simulink subsystem "BMS_slave"  (R2021a)
settings: Solver=VariableStepAuto  StartTime=0.0  StopTime=10.0  RelTol=1e-3
undefined symbols (not defined in the file): Discharge_Res
libraries: fl_lib x30, nesl_utility x20, ee_lib x10
settings Model: Creator=Carlo Edoardo  LastModifiedBy=Carlo Edoardo

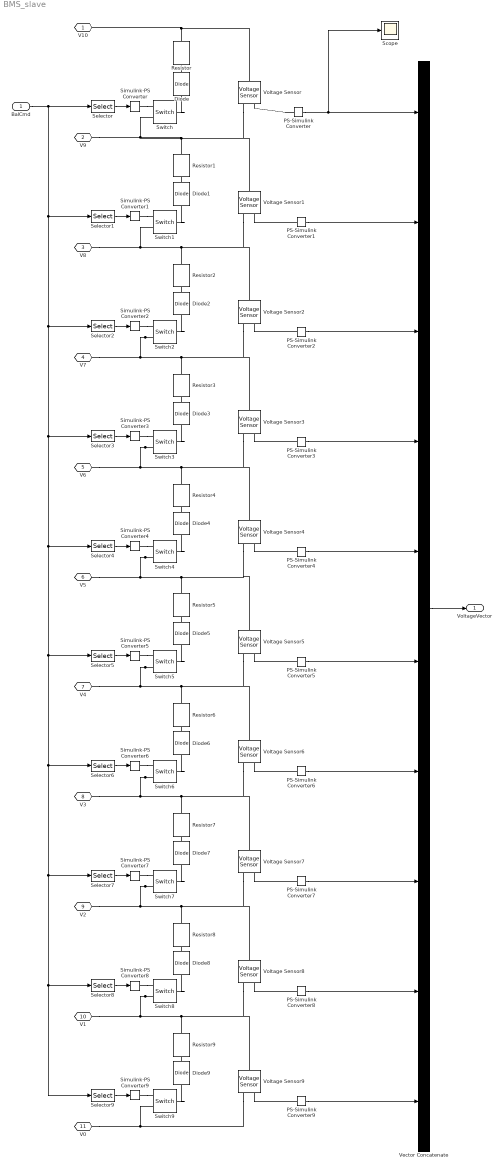
== system BMS_slave ==
  BalCmd : Inport
  Diode{,1..9} (10 alike) : ee_lib/Semiconductors & Converters/Diode  ModelType=ee.enum.diode.modelType.pwl  IfMat=[.07, .12, .19, 1.75, 4.24, 7.32, 11.2; .16, .3, .72, 2.14, 4.02, 6.35, 9.12] A  TjVec=[25, 125] degC  VfVec=[.5, .7, .9, 1.3, 1.7, 2.1, 2.5] V  Vf=0.6 V  Ron=0.3 Ohm  Goff=1e-8 S  prmExp=ee.enum.diode.expParam.useTwo  I12=[.0137, .545] A  V12=[.6, .7] V  IS=1e-12 A  ec=1  I1=0.0137 A  V1=0.6 V  RS=0 Ohm  Tmeas=25 degC  N_series=1  N_parallel=1  Rz=0.3 Ohm  BV=inf V  C_param=ee.enum.diode.capParam.fixed  CJ=5 pF  CJ0=5 pF  VJ=1 V  Mgrad=0.5  Vvec=[.1, 10, 100] V  Cvec=[3.5, 1, .4] pF  FC=0.5  Q_param=ee.enum.diode.recoveryParam.off  iRM=-7.15 A  iF=4 A  didt=-750 A/us  trr_factor=3  trr=115 ns  Qrr=150 s*nA  TT=50 ns  tau=100 ns  T_param=ee.enum.diode.temperatureParam.off  IS_T2=1.25e-7 A  I1_T2=0.245 A  V1_T2=0.5 V  Tmeas2=125 degC  EG_param=ee.enum.diode.egapParam.material_si  EG=1.11 eV  XTI_param=ee.enum.diode.xtiParam.pn  XTI=3  dBVdT=0 V/K  enable_faults=ee.enum.faults.faultEnable.no  fault_action=ee.enum.faults.faultAction.none  fault_types=ee.enum.diode.faults.open  tau_fault=1e-3 s  IfMat_faulted=[.07, .12, .19, 1.75, 4.24, 7.32, 11.2; .16, .3, .72, 2.14, 4.02, 6.35, 9.12] A  VfVec_faulted=[.5, .7, .9, 1.3, 1.7, 2.1, 2.5] V  Ropen_faulted=1000 Ohm  Gshort_faulted=1000 1/Ohm  Vf_faulted=0.6 V  Ron_faulted=0.3 Ohm  Goff_faulted=1e-8 S  I12_faulted=[.0137, .545] A  V12_faulted=[.6, .7] V  IS_faulted=1e-12 A  ec_faulted=1  I1_faulted=0.0137 A  V1_faulted=0.6 V  RS_faulted=0 Ohm  Rz_faulted=0.3 Ohm  BV_faulted=inf V  Cscale_faulted=100  enable_temporal_fault=ee.enum.faults.faultEnable.no  t_fault=inf s  enable_behavioral_fault=ee.enum.faults.faultEnable.no  max_permissible_voltage=inf V  n_fail_on_voltage=1  max_permissible_current=inf A  t_fail_on_current=1 s  max_permissible_dVdt=inf V/s  Tdevice=25 degC  i_specify=off  i_priority=None  i=0 A  i_nominal_specify=off  i_nominal_unit=A  i_nominal_value=1  v_specify=off  v_priority=None  v=0 V  v_nominal_specify=off  v_nominal_unit=V  v_nominal_value=1  i_diode_specify=off  i_diode_priority=None  i_diode=0 A  i_diode_nominal_specify=off  i_diode_nominal_unit=A  i_diode_nominal_value=1  v_diode_specify=off  v_diode_priority=None  v_diode=0 V  v_diode_nominal_specify=off  v_diode_nominal_unit=V  v_diode_nominal_value=1  i_capacitor_specify=off  i_capacitor_priority=None  i_capacitor=0 A  i_capacitor_nominal_specify=off  i_capacitor_nominal_unit=A  i_capacitor_nominal_value=1  v_capacitor_specify=off  v_capacitor_priority=None  v_capacitor=0 V  v_capacitor_nominal_specify=off  v_capacitor_nominal_unit=V  v_capacitor_nominal_value=1  power_dissipated_specify=off  power_dissipated_priority=None  power_dissipated=0 W  power_dissipated_nominal_specify=off  power_dissipated_nominal_unit=W  power_dissipated_nominal_value=1  max_permissible_temperature=inf K  t_fail_on_temperature=1 s  thermal_network_parameterization=ee.enum.thermalNetworkTopology.cauer  Rth=[0, 10] K/W  Rth_Foster=[4, 6] K/W  thermal_mass_parameterization=ee.enum.thermalNetwork.timeconstant  thermal_mass=[0, 1] J/K  thermal_mass_Foster=[1.5, 3] J/K  thermal_time_constant=[0, 10] s  thermal_time_constant_Foster=[6, 18] s  thermal_mass_initial_temperatures=[25, 25] degC
  PS-Simulink Converter{,1..9} (10 alike) : nesl_utility/PS-Simulink Converter  PhysicalDomain=network_engine_domain  SubClassName=ps_output  LeftPortType=input  RightPortType=output  PseudoPeriodic=off  Frequencies=[]  Unit=inherit  AffineConversion=off
      settings: SourceProductBaseCode=PW,SS
  Resistor{,1..9} (10 alike) : fl_lib/Electrical/Electrical Elements/Resistor  R=Discharge_Res Ohm  i_specify=off  i_priority=None  i=0 A  i_nominal_specify=off  i_nominal_unit=A  i_nominal_value=1  v_specify=off  v_priority=None  v=0 V  v_nominal_specify=off  v_nominal_unit=V  v_nominal_value=1
  Scope : Scope
  Selector : Selector  InputPortWidth=10  IndexOptions=Index vector (dialog)  Indices=1  OutputSizes=1
  Selector1 : Selector  InputPortWidth=10  IndexOptions=Index vector (dialog)  Indices=2  OutputSizes=1
  Selector2 : Selector  InputPortWidth=10  IndexOptions=Index vector (dialog)  Indices=3  OutputSizes=1
  Selector3 : Selector  InputPortWidth=10  IndexOptions=Index vector (dialog)  Indices=4  OutputSizes=1
  Selector4 : Selector  InputPortWidth=10  IndexOptions=Index vector (dialog)  Indices=5  OutputSizes=1
  Selector5 : Selector  InputPortWidth=10  IndexOptions=Index vector (dialog)  Indices=6  OutputSizes=1
  Selector6 : Selector  InputPortWidth=10  IndexOptions=Index vector (dialog)  Indices=7  OutputSizes=1
  Selector7 : Selector  InputPortWidth=10  IndexOptions=Index vector (dialog)  Indices=8  OutputSizes=1
  Selector8 : Selector  InputPortWidth=10  IndexOptions=Index vector (dialog)  Indices=9  OutputSizes=1
  Selector9 : Selector  InputPortWidth=10  IndexOptions=Index vector (dialog)  Indices=10  OutputSizes=1
  Simulink-PS Converter{,1..9} (10 alike) : nesl_utility/Simulink-PS Converter  PhysicalDomain=network_engine_domain  SubClassName=ps_input  LeftPortType=input  RightPortType=output  PseudoPeriodic=off  Frequencies=[]  NoiseDistribution=none  NoiseParameters=[]  Unit=1  AffineConversion=off  FilteringAndDerivatives=provide  SimscapeFilterOrder=1  InputFilterTimeConstant=0.001  UdotUserProvided=0
      settings: SourceProductBaseCode=PW,SS
  Switch{,1..9} (10 alike) : fl_lib/Electrical/Electrical Elements/Switch  R_closed=0.01 Ohm  G_open=1e-8 1/Ohm  Threshold=0.5  i_specify=off  i_priority=None  i=0 A  i_nominal_specify=off  i_nominal_unit=A  i_nominal_value=1  v_specify=off  v_priority=None  v=0 V  v_nominal_specify=off  v_nominal_unit=V  v_nominal_value=1
  Vector Concatenate : Concatenate  NumInputs=10
  Voltage Sensor{,1..9} (10 alike) : fl_lib/Electrical/Electrical Sensors/Voltage Sensor
  V10 : PMIOPort  Side=Left
  V9 : PMIOPort  Port=2  Side=Left
  V8 : PMIOPort  Port=3  Side=Left
  V7 : PMIOPort  Port=4  Side=Left
  V6 : PMIOPort  Port=5  Side=Left
  V5 : PMIOPort  Port=6  Side=Left
  V4 : PMIOPort  Port=7  Side=Left
  V3 : PMIOPort  Port=8  Side=Left
  V2 : PMIOPort  Port=9  Side=Left
  V1 : PMIOPort  Port=10  Side=Left
  V0 : PMIOPort  Port=11  Side=Left
  VoltageVector : Outport
  wires:
  Selector9/1 -> Simulink-PS Converter9/1
  Selector8/1 -> Simulink-PS Converter8/1
  Selector7/1 -> Simulink-PS Converter7/1
  Selector6/1 -> Simulink-PS Converter6/1
  Selector5/1 -> Simulink-PS Converter5/1
  Selector4/1 -> Simulink-PS Converter4/1
  Selector3/1 -> Simulink-PS Converter3/1
  Selector2/1 -> Simulink-PS Converter2/1
  Selector1/1 -> Simulink-PS Converter1/1
  Selector/1 -> Simulink-PS Converter/1
  BalCmd/1 -> Selector2/1, Selector3/1, Selector4/1, Selector5/1, Selector6/1, Selector7/1, Selector8/1, Selector9/1, Selector1/1, Selector/1
  Vector Concatenate/1 -> VoltageVector/1
  PS-Simulink Converter8/1 -> Vector Concatenate/9
  PS-Simulink Converter7/1 -> Vector Concatenate/8
  PS-Simulink Converter6/1 -> Vector Concatenate/7
  PS-Simulink Converter5/1 -> Vector Concatenate/6
  PS-Simulink Converter4/1 -> Vector Concatenate/5
  PS-Simulink Converter3/1 -> Vector Concatenate/4
  PS-Simulink Converter2/1 -> Vector Concatenate/3
  PS-Simulink Converter1/1 -> Vector Concatenate/2
  PS-Simulink Converter/1 -> Vector Concatenate/1, Scope/1
  PS-Simulink Converter9/1 -> Vector Concatenate/10
  connections:
  V0/RConn1 -- Switch9/RConn2 -- Voltage Sensor9/RConn2
  Switch8/RConn2 -- Resistor9/LConn1 -- Voltage Sensor9/LConn1 -- Voltage Sensor8/RConn2 -- V1/RConn1
  Switch7/RConn2 -- Resistor8/LConn1 -- Voltage Sensor8/LConn1 -- Voltage Sensor7/RConn2 -- V2/RConn1
  Switch6/RConn2 -- Resistor7/LConn1 -- Voltage Sensor7/LConn1 -- Voltage Sensor6/RConn2 -- V3/RConn1
  Switch5/RConn2 -- Resistor6/LConn1 -- Voltage Sensor6/LConn1 -- Voltage Sensor5/RConn2 -- V4/RConn1
  Switch4/RConn2 -- Resistor5/LConn1 -- Voltage Sensor5/LConn1 -- Voltage Sensor4/RConn2 -- V5/RConn1
  Switch3/RConn2 -- Resistor4/LConn1 -- Voltage Sensor4/LConn1 -- Voltage Sensor3/RConn2 -- V6/RConn1
  Switch2/RConn2 -- Resistor3/LConn1 -- Voltage Sensor3/LConn1 -- Voltage Sensor2/RConn2 -- V7/RConn1
  V8/RConn1 -- Switch1/RConn2 -- Resistor2/LConn1 -- Voltage Sensor2/LConn1 -- Voltage Sensor1/RConn2
  V9/RConn1 -- Switch/RConn2 -- Resistor1/LConn1 -- Voltage Sensor1/LConn1 -- Voltage Sensor/RConn2
  Voltage Sensor/LConn1 -- Resistor/LConn1 -- V10/RConn1
  Simulink-PS Converter9/RConn1 -- Switch9/RConn1
  Simulink-PS Converter8/RConn1 -- Switch8/RConn1
  Simulink-PS Converter7/RConn1 -- Switch7/RConn1
  Simulink-PS Converter6/RConn1 -- Switch6/RConn1
  Simulink-PS Converter5/RConn1 -- Switch5/RConn1
  Simulink-PS Converter4/RConn1 -- Switch4/RConn1
  Simulink-PS Converter3/RConn1 -- Switch3/RConn1
  Simulink-PS Converter2/RConn1 -- Switch2/RConn1
  Simulink-PS Converter1/RConn1 -- Switch1/RConn1
  Simulink-PS Converter/RConn1 -- Switch/RConn1
  Voltage Sensor9/RConn1 -- PS-Simulink Converter9/LConn1
  Voltage Sensor8/RConn1 -- PS-Simulink Converter8/LConn1
  Voltage Sensor7/RConn1 -- PS-Simulink Converter7/LConn1
  Voltage Sensor6/RConn1 -- PS-Simulink Converter6/LConn1
  Voltage Sensor5/RConn1 -- PS-Simulink Converter5/LConn1
  Voltage Sensor4/RConn1 -- PS-Simulink Converter4/LConn1
  Voltage Sensor3/RConn1 -- PS-Simulink Converter3/LConn1
  Voltage Sensor2/RConn1 -- PS-Simulink Converter2/LConn1
  Voltage Sensor1/RConn1 -- PS-Simulink Converter1/LConn1
  PS-Simulink Converter/LConn1 -- Voltage Sensor/RConn1
  Switch9/LConn1 -- Diode9/RConn1
  Resistor9/RConn1 -- Diode9/LConn1
  Switch8/LConn1 -- Diode8/RConn1
  Resistor8/RConn1 -- Diode8/LConn1
  Switch7/LConn1 -- Diode7/RConn1
  Resistor7/RConn1 -- Diode7/LConn1
  Switch6/LConn1 -- Diode6/RConn1
  Resistor6/RConn1 -- Diode6/LConn1
  Switch5/LConn1 -- Diode5/RConn1
  Resistor5/RConn1 -- Diode5/LConn1
  Switch4/LConn1 -- Diode4/RConn1
  Resistor4/RConn1 -- Diode4/LConn1
  Switch3/LConn1 -- Diode3/RConn1
  Resistor3/RConn1 -- Diode3/LConn1
  Switch2/LConn1 -- Diode2/RConn1
  Resistor2/RConn1 -- Diode2/LConn1
  Diode1/LConn1 -- Resistor1/RConn1
  Switch1/LConn1 -- Diode1/RConn1
  Switch/LConn1 -- Diode/RConn1
  Diode/LConn1 -- Resistor/RConn1
